simulink model "Ahmad_Fares_Kalman"  (Simulink 5.0)
settings: Solver=ode1  SolverMode=SingleTasking  StartTime=0.0  StopTime=120.0  FixedStep=0.001  RelTol=1e-3
libraries: pci1711 x3
CloseFcn:
  | rtwprivate ssgencode ModelCloseRequest InvertedPD
settings Model: LastModifiedBy=yousef  ExtModeMexFile=rtwinext  ExtModeTrigMode=oneshot  ExtModeTrigDuration=100000  ExtModeLogAll=off  SimulationMode=external  LimitDataPoints=off  BlockReductionOpt=off  BooleanDataType=off  RTWSystemTargetFile=rtwinfbk.tlc  RTWTemplateMakefile=winfbktmf  RTWOptions="-aCCOptimize=1 -aEnforceIntegerDowncast=1 -aExtMode=1 -aFoldNonRolledExpr=1 -aForceParamTrailComments=0 -aGenerateComments=1 -aGenerateReport=0 -aIncDataTypeInIds=0 -aIncHierarchyInIds=0 -aInlineInvariantSignals=0 -aInlineParameters=0 -aInlinedPrmAccess=\"Literals\" -aLocalBlockOutputs=1 -aMaxRTWIdLen=31 -aPrefixModelToSubsysFcnNames=1 -aRTWVerbose=1 -aRebuildAll=0 -aRollThreshold=5 -aShowEliminatedStatements=1"

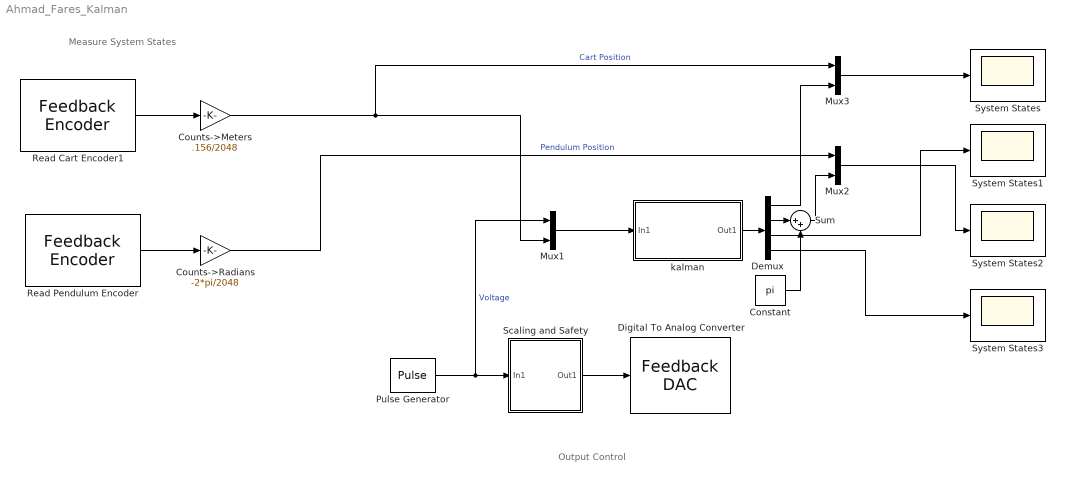
== system Ahmad_Fares_Kalman ==
  note: Measure System States
  note: Output Control
  Constant : Constant  Value=pi
  Counts->Meters : Gain  Gain=.156/2048  SaturateOnIntegerOverflow=on
  Counts->Radians : Gain  Gain=-2*pi/2048  SaturateOnIntegerOverflow=on
  Demux : Demux
  Digital To Analog Converter : pci1711/Advantech  PCI1711 I//O Board Lib/Feedback DAC  channel=0  range=0  tsamp=0.001  hwAccess=on
  Mux1 : Mux  Inputs=2
  Mux2 : Mux  Inputs=2
  Mux3 : Mux  Inputs=2
  Pulse Generator : DiscretePulseGenerator  PulseType=Time based  Amplitude=1.2  Period=100  PulseWidth=0.5  PhaseDelay=20  VectorParams1D=off
  Read Cart Encoder1 : pci1711/Advantech  PCI1711 I//O Board Lib/Feedback Encoder   channel=0  offset=0  tsamp=0.001  hwAccess=on
  Read Pendulum Encoder : pci1711/Advantech  PCI1711 I//O Board Lib/Feedback Encoder   channel=1  offset=-1024  tsamp=0.001  hwAccess=on
  Scaling and Safety : Subsystem
  Sum : Sum  Inputs=|++  SaturateOnIntegerOverflow=on
  System States{,1..3} (4 alike) : Scope
      System States settings: TimeRange=50  YMin=0.2802  YMax=0.280575  SaveName=y  Decimation=0.1  SampleInput=on  SampleTime=0.01
      System States1 settings: TimeRange=50  YMin=-0.4  YMax=0.4  SaveName=y1  Decimation=0.1  SampleInput=on  SampleTime=0.01
      System States2 settings: TimeRange=50  YMin=-2.5e+301  YMax=5e+302  SaveName=y2  Decimation=0.1  SampleInput=on  SampleTime=0.01
      System States3 settings: TimeRange=50  YMin=-0.125  YMax=0.025  SaveName=y3  Decimation=0.1  SampleInput=on  SampleTime=0.01
  kalman : Subsystem  mask{Q=[1e-03 1e-03 1000 1], R=1e-04}
      mask init:
      | mc = 1.12;
      | mpw = 0.095;
      | mps = 0.025;
      | l = 0.033245968; % 0.0167903;
      | fc = 2.53165; % FS = 2.53165; FC = 2.28133
      | fp = 0.000107443;
      | J = 0.013935418; % 0.0135735;
      | g = 9.81;
      | vf = 9.4/2.5; % Voltage to Motor Force ratio % 17.463
      | mp = mpw + mps;
      | a = l^2 + J/(mc + mp);
      | mu = (mc + mp)*l;
      | Ts = 0.01;
      | 
      | % theta 0 in upward position
      | % theta pi in downward position
      | s = -1; % 1 when upward  -1 when downward
      | 
      | A = [0          0              1               0;
      |      0          0              0               1;
      |      0      (l*mu*g)/J    -(a*fc)/J    -(l*fp)/J;
      |      0      s*(mu*g)/J    -s*(l*fc)/J    -(fp)/J];
      |  
      | B = [           0;
      |                 0;
      |          (vf*a)/J;
      |       (s*vf*l)/J];
      |   
      | C = [1 0 0 0];
      |  
      | D = [0];
      | 
      | G = ones(4,4);
      | % H = 1;
      | 
      | sys = ss(A,[B G],[C],[D zeros(1,4)]); % continous sys
      | % sysd = c2d(sys,Ts);
      | 
      | % Ad = [Ts*A + eye(4)];
      | % Bd = Ts*B;
      | 
      | Qn = diag(Q);
      | Rn = diag(R);
      | 
      | [kf,L,P] = kalman(sys,Qn,Rn);
      | 
      | Ak = A - L*C;
      | Bk = [B L];
      | Ck = eye(4);
      | Dk = 0*[B L];
  wires:
  Counts->Meters/1 -> Mux1/2, Mux3/1  "Cart Position"
  Counts->Radians/1 -> Mux2/1  "Pendulum Position"
  Scaling and Safety/1(Out1) -> Digital To Analog Converter/1
  Read Cart Encoder1/1 -> Counts->Meters/1
  Read Pendulum Encoder/1 -> Counts->Radians/1
  Mux1/1 -> kalman/1(In1)
  kalman/1(Out1) -> Demux/1
  Pulse Generator/1 -> Scaling and Safety/1(In1), Mux1/1  "Voltage"
  Demux/1 -> Mux3/2
  Mux3/1 -> System States/1
  Demux/3 -> System States1/1
  Demux/4 -> System States3/1
  Constant/1 -> Sum/2
  Demux/2 -> Sum/1
  Sum/1 -> Mux2/2
  Mux2/1 -> System States2/1

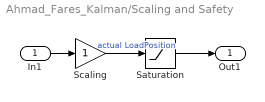
== system Ahmad_Fares_Kalman/Scaling and Safety ==
  In1 : Inport
  Saturation : Saturate  UpperLimit=2.5  LowerLimit=-2.5
  Scaling : Gain  SaturateOnIntegerOverflow=on
  Out1 : Outport
  wires:
  Saturation/1 -> Out1/1
  In1/1 -> Scaling/1
  Scaling/1 -> Saturation/1  "actual LoadPosition"

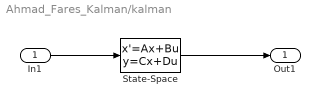
== system Ahmad_Fares_Kalman/kalman ==
  In1 : Inport
  State-Space : StateSpace  A=Ak  B=Bk  C=Ck  D=Dk
  Out1 : Outport
  wires:
  In1/1 -> State-Space/1
  State-Space/1 -> Out1/1
